simulink model "FW_TFLateralModel"  (R2020a)
settings: Solver=ode45  StartTime=0.0  StopTime=Trun  RelTol=1e-3  EnableMultiTasking=on
undefined symbols (not defined in the file): a_phi1, a_phi2
settings Model: Creator=user  LastModifiedBy=patel
settings DataIOCC: LimitDataPoints=on  SaveFormat=Array  ReturnWorkspaceOutputs=off
settings OptimizationCC: LifeSpan=inf
settings DebuggingCC: SFUnexpectedBacktrackingDiag=warning  SFNoUnconditionalDefaultTransitionDiag=warning  SFExecutionAtInitializationDiag=none  ArithmeticOperatorsInVariantConditions=warning
settings HardwareCC: ProdBitPerPointer=32  ProdBitPerSizeT=32  ProdBitPerPtrDiffT=32  ProdLargestAtomicFloat=None  ProdIntDivRoundTo=Undefined  ProdEndianess=Unspecified  ProdWordSize=32  ProdHWDeviceType=32-bit Generic
settings ModelReferenceCC: PropagateSignalLabelsOutOfModel=off
settings SFSimCC: SimUseLocalCustomCode=off  CustomCodeUndefinedFunction=UseInterfaceOnly
settings RTWCC: RTWUseLocalCustomCode=off
settings CodeAppCC: StateflowObjectComments=on
settings GRTTargetCC: TargetLangStandard=C89/C90 (ANSI)
settings ConfigComp: CovMetricSettings=dw  CovHtmlReporting=on  CovSaveCumulativeToWorkspaceVar=on  CovSaveSingleToWorkspaceVar=on  CovExternalEMLEnable=off

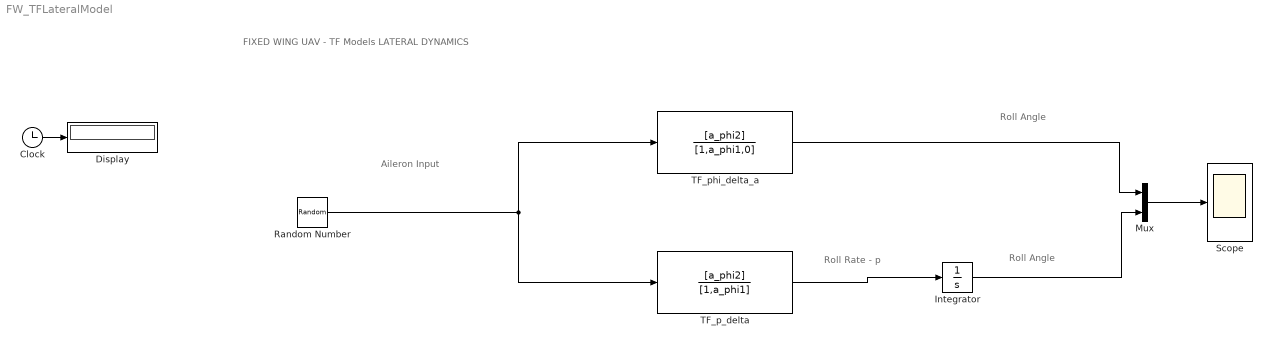
== system FW_TFLateralModel ==
  note: Roll Angle
  note: Roll Rate - p
  note: Roll Angle
  note: Aileron Input
  note: FIXED WING UAV - TF Models LATERAL DYNAMICS
  Clock : Clock
  Display : Display
  Integrator : Integrator
  Mux : Mux  Inputs=2
  Random Number : RandomNumber  SampleTime=0.1
  Scope : Scope
  TF_p_delta : TransferFcn  Numerator=[a_phi2]  Denominator=[1,a_phi1]
  TF_phi_delta_a : TransferFcn  Numerator=[a_phi2]  Denominator=[1,a_phi1,0]
  wires:
  TF_p_delta/1 -> Integrator/1
  Random Number/1 -> TF_phi_delta_a/1, TF_p_delta/1
  TF_phi_delta_a/1 -> Mux/1
  Integrator/1 -> Mux/2
  Mux/1 -> Scope/1
  Clock/1 -> Display/1
